simulink model "F16_Model"  (R2023b)
settings: Solver=ode4  StartTime=0.0  StopTime=inf  FixedStep=deltaTime  RelTol=1e-3
PreLoadFcn:
  | addpath(genpath(cd))
InitFcn:
  | Run_Config
undefined symbols (not defined in the file or in its folder): controlDeflections, dataBase, deltaLEF, statesFinal
libraries: simulink_extras x17, vrlib x1, sharedtransform x1
(part 2 of 2)

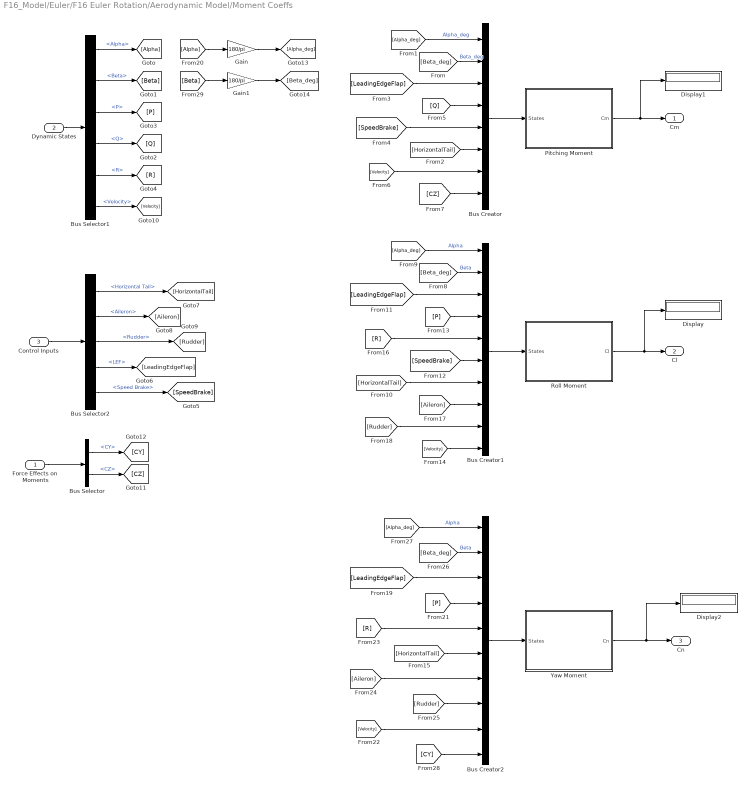
== system F16_Model/Euler/F16 Euler Rotation/Aerodynamic Model/Moment Coeffs ==
  Force Effects on Moments : Inport
  Dynamic States : Inport  Port=2
  Control Inputs : Inport  Port=3
  Bus Creator : BusCreator  Inputs=8
  Bus Creator1 : BusCreator  Inputs=10
  Bus Creator2 : BusCreator  Inputs=10
  Bus Selector : BusSelector  OutputSignals=CY,CZ
  Bus Selector1 : BusSelector  OutputSignals=Alpha,Beta,P,Q,R,Velocity
  Bus Selector2 : BusSelector  OutputSignals=Horizontal Tail,Aileron,Rudder,LEF,Speed Brake
  Display : Display
  Display1 : Display
  Display2 : Display
  Gain : Gain  Gain=180/pi
  Gain1 : Gain  Gain=180/pi
  Pitching Moment : Subsystem
  Roll Moment : Subsystem
  Yaw Moment : Subsystem
  " Cm" : Outport
  " Cl" : Outport  Port=2
  " Cn" : Outport  Port=3
  wires:
  Pitching Moment/1(Cm) -> Display1/1, " Cm"/1
  Bus Creator/1 -> Pitching Moment/1(States)
  [SpeedBrake] -> Bus Creator/5
  [LeadingEdgeFlap] -> Bus Creator/3
  [Q] -> Bus Creator/4
  [HorizontalTail] -> Bus Creator/6
  [Velocity] -> Bus Creator/7
  [CZ] -> Bus Creator/8
  Force Effects on Moments/1 -> Bus Selector/1
  Bus Selector/1 -> [CY]  "<CY>"
  Bus Selector/2 -> [CZ]  "<CZ>"
  [P] -> Bus Creator1/4
  [LeadingEdgeFlap] -> Bus Creator1/3
  Roll Moment/1(Cl) -> Display/1, " Cl"/1
  Yaw Moment/1(Cn) -> Display2/1, " Cn"/1
  [Velocity] -> Bus Creator1/10
  [R] -> Bus Creator1/5
  [SpeedBrake] -> Bus Creator1/6
  [HorizontalTail] -> Bus Creator1/7
  [Aileron] -> Bus Creator1/8
  [Rudder] -> Bus Creator1/9
  [Rudder] -> Bus Creator2/8
  [Aileron] -> Bus Creator2/7
  [HorizontalTail] -> Bus Creator2/6
  [R] -> Bus Creator2/5
  [Velocity] -> Bus Creator2/9
  [LeadingEdgeFlap] -> Bus Creator2/3
  [P] -> Bus Creator2/4
  Bus Creator2/1 -> Yaw Moment/1(States)
  Bus Selector1/4 -> [Q]  "<Q>"
  Bus Selector2/1 -> [HorizontalTail]  "<Horizontal Tail>"
  Control Inputs/1 -> Bus Selector2/1
  Bus Selector2/5 -> [SpeedBrake]  "<Speed Brake>"
  Bus Selector2/2 -> [Aileron]  "<Aileron>"
  Bus Selector1/6 -> [Velocity]  "<Velocity>"
  Bus Selector1/3 -> [P]  "<P>"
  Bus Selector1/2 -> [Beta]  "<Beta>"
  Bus Selector2/3 -> [Rudder]  "<Rudder>"
  Bus Selector1/5 -> [R]  "<R>"
  Bus Selector2/4 -> [LeadingEdgeFlap]  "<LEF>"
  Dynamic States/1 -> Bus Selector1/1
  Bus Selector1/1 -> [Alpha]  "<Alpha>"
  Bus Creator1/1 -> Roll Moment/1(States)
  Gain1/1 -> [Beta_deg]
  [Beta] -> Gain1/1
  [Alpha] -> Gain/1
  Gain/1 -> [Alpha_deg]
  [Alpha_deg] -> Bus Creator/1  "Alpha_deg"
  [Beta_deg] -> Bus Creator/2  "Beta_deg"
  [Alpha_deg] -> Bus Creator1/1  "Alpha"
  [Beta_deg] -> Bus Creator1/2  "Beta"
  [Alpha_deg] -> Bus Creator2/1  "Alpha"
  [Beta_deg] -> Bus Creator2/2  "Beta"
  [CY] -> Bus Creator2/10

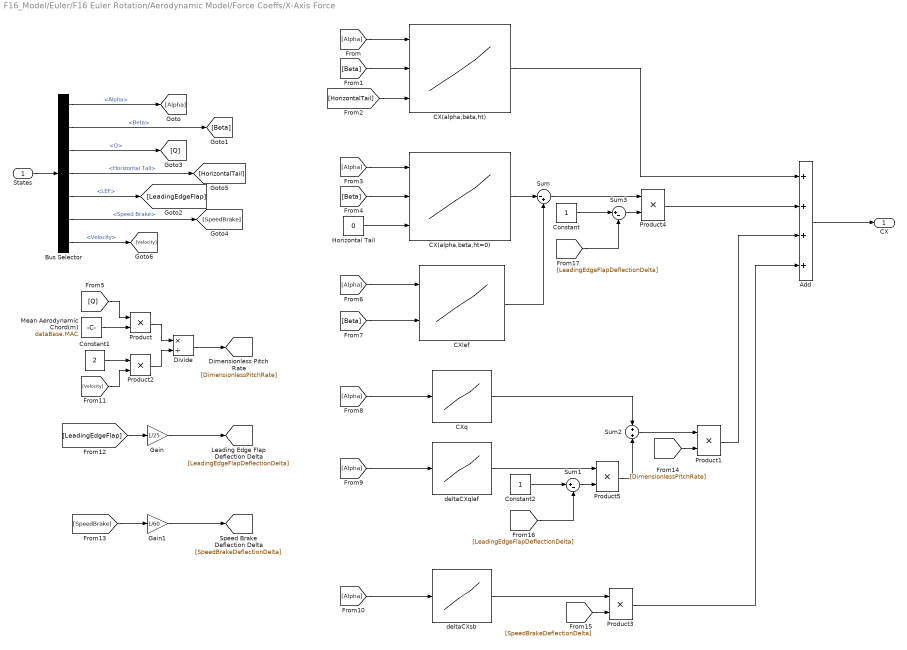
== system F16_Model/Euler/F16 Euler Rotation/Aerodynamic Model/Force Coeffs/X-Axis Force ==
  States : Inport
  Add : Sum  Inputs=++++
  Bus Selector : BusSelector  OutputSignals=Alpha,Beta,Q,Horizontal Tail,LEF,Speed Brake,Velocity
  CX(alpha,beta,ht) : Lookup_n-D  NumberOfTableDimensions=3  BreakpointsForDimension1=dataBase.f16_AerodynamicData.BP.CX.CX.alpha  BreakpointsForDimension2=dataBase.f16_AerodynamicData.BP.CX.CX.beta  BreakpointsForDimension3=dataBase.f16_AerodynamicData.BP.CX.CX.dHT  Table=dataBase.f16_AerodynamicData.data.CX.CX  InternalRulePriority=Speed  RndMeth=Simplest
      settings: InputPortMap=u0,u1,u2
  CX(alpha,beta,ht=0) : Lookup_n-D  NumberOfTableDimensions=3  BreakpointsForDimension1=dataBase.f16_AerodynamicData.BP.CX.CX.alpha  BreakpointsForDimension2=dataBase.f16_AerodynamicData.BP.CX.CX.beta  BreakpointsForDimension3=dataBase.f16_AerodynamicData.BP.CX.CX.dHT  Table=dataBase.f16_AerodynamicData.data.CX.CX  InternalRulePriority=Speed  RndMeth=Simplest
      settings: InputPortMap=u0,u1,u2
  CXlef : Lookup_n-D  BreakpointsForDimension1=dataBase.f16_AerodynamicData.BP.CX.CXlef.alpha  BreakpointsForDimension2=dataBase.f16_AerodynamicData.BP.CX.CXlef.beta  Table=dataBase.f16_AerodynamicData.data.CX.CXlef  InternalRulePriority=Speed  RndMeth=Simplest
      settings: InputPortMap=u0,u1
  CXq : Lookup_n-D  NumberOfTableDimensions=1  BreakpointsForDimension1=dataBase.f16_AerodynamicData.BP.CX.CXq.alpha  Table=dataBase.f16_AerodynamicData.data.CX.CXq  InternalRulePriority=Speed  RndMeth=Simplest
  Constant : Constant
  Constant1 : Constant  Value=2
  Constant2 : Constant
  Divide : Product  Inputs=*/
  Gain : Gain  Gain=1/25
  Gain1 : Gain  Gain=1/60
  Horizontal Tail : Constant  Value=0
  Mean Aerodynamic Chord(m) : Constant  Value=dataBase.MAC
  Product{,1..5} (6 alike) : Product
  Sum : Sum  Inputs=|-+
  Sum1 : Sum  Inputs=|+-
  Sum2 : Sum  Inputs=+|+
  Sum3 : Sum  Inputs=|+-
  deltaCXqlef : Lookup_n-D  NumberOfTableDimensions=1  BreakpointsForDimension1=dataBase.f16_AerodynamicData.BP.CX.deltaCXqlef.alpha  Table=dataBase.f16_AerodynamicData.data.CX.deltaCXqlef  InternalRulePriority=Speed  RndMeth=Simplest
  deltaCXsb : Lookup_n-D  NumberOfTableDimensions=1  BreakpointsForDimension1=dataBase.f16_AerodynamicData.BP.CX.deltaCXSB.alpha  Table=dataBase.f16_AerodynamicData.data.CX.deltaCXSB  InternalRulePriority=Speed  RndMeth=Simplest
  CX : Outport  VectorParamsAs1DForOutWhenUnconnected=off
  wires:
  States/1 -> Bus Selector/1
  [Alpha] -> CX(alpha,beta,ht)/1
  [Beta] -> CX(alpha,beta,ht)/2
  [HorizontalTail] -> CX(alpha,beta,ht)/3
  [Alpha] -> CX(alpha,beta,ht=0)/1
  Horizontal Tail/1 -> CX(alpha,beta,ht=0)/3
  [Beta] -> CX(alpha,beta,ht=0)/2
  CX(alpha,beta,ht=0)/1 -> Sum/1
  CXlef/1 -> Sum/2
  [Alpha] -> CXlef/1
  [Beta] -> CXlef/2
  [Alpha] -> CXq/1
  [Alpha] -> deltaCXqlef/1
  [Alpha] -> deltaCXsb/1
  [Q] -> Product/1
  Mean Aerodynamic Chord(m)/1 -> Product/2
  Product/1 -> Divide/1
  Divide/1 -> [DimensionlessPitchRate]
  Add/1 -> CX/1
  CX(alpha,beta,ht)/1 -> Add/1
  [LeadingEdgeFlap] -> Gain/1
  [SpeedBrake] -> Gain1/1
  Gain1/1 -> [SpeedBrakeDeflectionDelta]
  CXq/1 -> Sum2/1
  Sum2/1 -> Product1/1
  Constant1/1 -> Product2/1
  [Velocity] -> Product2/2
  Product2/1 -> Divide/2
  [DimensionlessPitchRate] -> Product1/2
  deltaCXsb/1 -> Product3/1
  [SpeedBrakeDeflectionDelta] -> Product3/2
  Product1/1 -> Add/3
  Product3/1 -> Add/4
  Sum/1 -> Product4/1
  Product4/1 -> Add/2
  Gain/1 -> [LeadingEdgeFlapDeflectionDelta]
  Constant/1 -> Sum3/1
  Sum3/1 -> Product4/2
  [LeadingEdgeFlapDeflectionDelta] -> Sum3/2
  [LeadingEdgeFlapDeflectionDelta] -> Sum1/2
  Constant2/1 -> Sum1/1
  Product5/1 -> Sum2/2
  deltaCXqlef/1 -> Product5/1
  Sum1/1 -> Product5/2
  Bus Selector/1 -> [Alpha]  "<Alpha>"
  Bus Selector/2 -> [Beta]  "<Beta>"
  Bus Selector/3 -> [Q]  "<Q>"
  Bus Selector/4 -> [HorizontalTail]  "<Horizontal Tail>"
  Bus Selector/5 -> [LeadingEdgeFlap]  "<LEF>"
  Bus Selector/6 -> [SpeedBrake]  "<Speed Brake>"
  Bus Selector/7 -> [Velocity]  "<Velocity>"

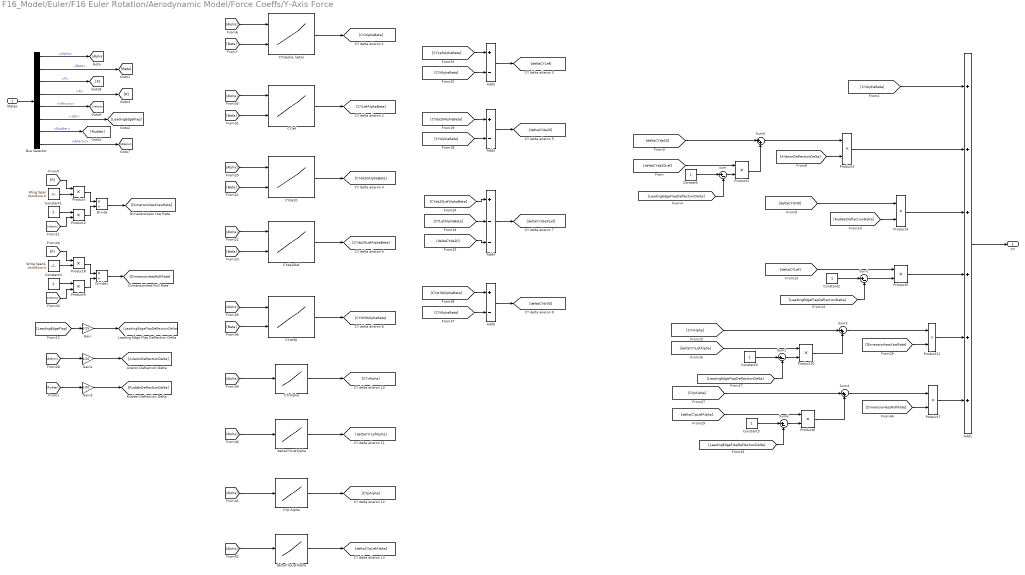
== system F16_Model/Euler/F16 Euler Rotation/Aerodynamic Model/Force Coeffs/Y-Axis Force ==
  States : Inport
  Add1 : Sum  Inputs=++++++
  Add2 : Sum  Inputs=+-
  Add3 : Sum  Inputs=+-
  Add4 : Sum  Inputs=+--
  Add5 : Sum  Inputs=+-
  Bus Selector : BusSelector  OutputSignals=Alpha,Beta,P,R,Velocity,LEF,Rudder,Aileron
  "CY(alpha, beta)" : Lookup_n-D  BreakpointsForDimension1=dataBase.f16_AerodynamicData.BP.CY.CY.alpha  BreakpointsForDimension2=dataBase.f16_AerodynamicData.BP.CY.CY.beta  Table=dataBase.f16_AerodynamicData.data.CY.CY  InternalRulePriority=Speed  RndMeth=Simplest
      settings: InputPortMap=u0,u1
  CYda20 : Lookup_n-D  BreakpointsForDimension1=dataBase.f16_AerodynamicData.BP.CY.CYda20.alpha  BreakpointsForDimension2=dataBase.f16_AerodynamicData.BP.CY.CYda20.beta  Table=dataBase.f16_AerodynamicData.data.CY.CYda20  InternalRulePriority=Speed  RndMeth=Simplest
      settings: InputPortMap=u0,u1
  CYda20lef : Lookup_n-D  BreakpointsForDimension1=dataBase.f16_AerodynamicData.BP.CY.CYda20lef.alpha  BreakpointsForDimension2=dataBase.f16_AerodynamicData.BP.CY.CYda20lef.beta  Table=dataBase.f16_AerodynamicData.data.CY.CYda20lef  InternalRulePriority=Speed  RndMeth=Simplest
      settings: InputPortMap=u0,u1
  CYdr30 : Lookup_n-D  BreakpointsForDimension1=dataBase.f16_AerodynamicData.BP.CY.CYdr30.alpha  BreakpointsForDimension2=dataBase.f16_AerodynamicData.BP.CY.CYdr30.beta  Table=dataBase.f16_AerodynamicData.data.CY.CYdr30  InternalRulePriority=Speed  RndMeth=Simplest
      settings: InputPortMap=u0,u1
  CYlef : Lookup_n-D  BreakpointsForDimension1=dataBase.f16_AerodynamicData.BP.CY.CYlef.alpha  BreakpointsForDimension2=dataBase.f16_AerodynamicData.BP.CY.CYlef.beta  Table=dataBase.f16_AerodynamicData.data.CY.CYlef  InternalRulePriority=Speed  RndMeth=Simplest
      settings: InputPortMap=u0,u1
  CYp Alpha : Lookup_n-D  NumberOfTableDimensions=1  BreakpointsForDimension1=dataBase.f16_AerodynamicData.BP.CY.CYp.alpha  Table=dataBase.f16_AerodynamicData.data.CY.CYp  InternalRulePriority=Speed  RndMeth=Simplest
  CYrAlpha : Lookup_n-D  NumberOfTableDimensions=1  BreakpointsForDimension1=dataBase.f16_AerodynamicData.BP.CY.CYr.alpha  Table=dataBase.f16_AerodynamicData.data.CY.CYr  InternalRulePriority=Speed  RndMeth=Simplest
  Constant{,2..3,5} (4 alike) : Constant
  Constant1 : Constant  Value=2
  Constant4 : Constant  Value=2
  Divide : Product  Inputs=*/
  Divide1 : Product  Inputs=*/
  Gain : Gain  Gain=1/25
  Gain2 : Gain  Gain=1/20
  Gain3 : Gain  Gain=1/30
  Product{,1..11} (12 alike) : Product
  Sum{,1..2,6} (4 alike) : Sum  Inputs=|+-
  Sum3 : Sum  Inputs=|++
  Sum4 : Sum  Inputs=|++
  Sum5 : Sum  Inputs=|++
  Wing Span : Constant  Value=dataBase.b
  Wing Span1 : Constant  Value=dataBase.b
  deltaCYpLefAlpha : Lookup_n-D  NumberOfTableDimensions=1  BreakpointsForDimension1=dataBase.f16_AerodynamicData.BP.CY.deltaCYplef.alpha  Table=dataBase.f16_AerodynamicData.data.CY.deltaCYplef  InternalRulePriority=Speed  RndMeth=Simplest
  deltaCYrLefAlpha : Lookup_n-D  NumberOfTableDimensions=1  BreakpointsForDimension1=dataBase.f16_AerodynamicData.BP.CY.deltaCYrlef.alpha  Table=dataBase.f16_AerodynamicData.data.CY.deltaCYrlef  InternalRulePriority=Speed  RndMeth=Simplest
  CY : Outport  VectorParamsAs1DForOutWhenUnconnected=off
  wires:
  Wing Span/1 -> Product/2
  Divide/1 -> [DimensionlessYawRate]
  [LeadingEdgeFlap] -> Gain/1
  Constant1/1 -> Product2/1
  [Beta] -> "CY(alpha, beta)"/2
  [R] -> Product/1
  States/1 -> Bus Selector/1
  Product2/1 -> Divide/2
  Product/1 -> Divide/1
  [Alpha] -> "CY(alpha, beta)"/1
  Gain/1 -> [LeadingEdgeFlapDeflectionDelta]
  [Velocity] -> Product2/2
  Add1/1 -> CY/1
  "CY(alpha, beta)"/1 -> [CYAlphaBeta]
  [Beta] -> CYda20/2
  [Alpha] -> CYda20/1
  [Alpha] -> CYda20lef/1
  [Beta] -> CYda20lef/2
  [Aileron] -> Gain2/1
  Gain2/1 -> [AileronDeflectionDelta]
  [Alpha] -> CYlef/1
  [Beta] -> CYlef/2
  CYlef/1 -> [CYLefAlphaBeta]
  Add2/1 -> [deltaCYLef]
  [CYAlphaBeta] -> Add2/2
  [CYLefAlphaBeta] -> Add2/1
  CYda20/1 -> [CYda20AlphaBeta]
  [CYda20AlphaBeta] -> Add3/1
  [CYAlphaBeta] -> Add3/2
  Add3/1 -> [deltaCYda20]
  CYda20lef/1 -> [CYda20LefAlphaBeta]
  [CYda20LefAlphaBeta] -> Add4/1
  [CYLefAlphaBeta] -> Add4/2
  [deltaCYda20] -> Add4/3
  Add4/1 -> [deltaCYda20Lef]
  CYdr30/1 -> [CYdr30AlphaBeta]
  [Alpha] -> CYdr30/1
  [Beta] -> CYdr30/2
  Add5/1 -> [deltaCYdr30]
  [CYAlphaBeta] -> Add5/2
  [CYdr30AlphaBeta] -> Add5/1
  [Alpha] -> CYrAlpha/1
  CYrAlpha/1 -> [CYrAlpha]
  deltaCYrLefAlpha/1 -> [deltaCYrLefAlpha]
  [Alpha] -> deltaCYrLefAlpha/1
  [Alpha] -> deltaCYpLefAlpha/1
  deltaCYpLefAlpha/1 -> [deltaCYpLefAlpha]
  CYp Alpha/1 -> [CYpAlpha]
  [Alpha] -> CYp Alpha/1
  [Velocity] -> Product9/2
  Product8/1 -> Divide1/1
  Product9/1 -> Divide1/2
  [P] -> Product8/1
  Constant4/1 -> Product9/1
  Divide1/1 -> [DimensionlessRollRate]
  Wing Span1/1 -> Product8/2
  Gain3/1 -> [RudderDeflectionDelta]
  [Rudder] -> Gain3/1
  [CYAlphaBeta] -> Add1/1
  [deltaCYda20Lef] -> Product1/1
  [deltaCYda20] -> Sum5/1
  Product1/1 -> Sum5/2
  Sum5/1 -> Product3/1
  [AileronDeflectionDelta] -> Product3/2
  Product3/1 -> Add1/2
  [RudderDeflectionDelta] -> Product4/2
  [deltaCYdr30] -> Product4/1
  Product4/1 -> Add1/3
  [deltaCYLef] -> Product5/1
  Product5/1 -> Add1/4
  [CYrAlpha] -> Sum3/1
  [deltaCYrLefAlpha] -> Product10/1
  Product10/1 -> Sum3/2
  [DimensionlessYawRate] -> Product11/2
  Sum3/1 -> Product11/1
  Product11/1 -> Add1/5
  Product7/1 -> Add1/6
  Sum4/1 -> Product7/1
  [DimensionlessRollRate] -> Product7/2
  Product6/1 -> Sum4/2
  [deltaCYpLefAlpha] -> Product6/1
  [CYpAlpha] -> Sum4/1
  Constant/1 -> Sum/1
  [LeadingEdgeFlapDeflectionDelta] -> Sum/2
  Sum/1 -> Product1/2
  Constant2/1 -> Sum1/1
  [LeadingEdgeFlapDeflectionDelta] -> Sum1/2
  Sum1/1 -> Product5/2
  Constant3/1 -> Sum2/1
  [LeadingEdgeFlapDeflectionDelta] -> Sum2/2
  Sum2/1 -> Product10/2
  Constant5/1 -> Sum6/1
  [LeadingEdgeFlapDeflectionDelta] -> Sum6/2
  Sum6/1 -> Product6/2
  Bus Selector/1 -> [Alpha]  "<Alpha>"
  Bus Selector/2 -> [Beta]  "<Beta>"
  Bus Selector/3 -> [P]  "<P>"
  Bus Selector/4 -> [R]  "<R>"
  Bus Selector/5 -> [Velocity]  "<Velocity>"
  Bus Selector/6 -> [LeadingEdgeFlap]  "<LEF>"
  Bus Selector/7 -> [Rudder]  "<Rudder>"
  Bus Selector/8 -> [Aileron]  "<Aileron>"

== system F16_Model/Euler/F16 Euler Rotation/Aerodynamic Model/Force Coeffs/Z-Axis Force ==
  States : Inport
  Add : Sum  Inputs=++++
  Bus Selector : BusSelector  OutputSignals=Alpha,Beta,Q,Horizontal Tail,LEF,Speed Brake,Velocity
  CZ(alpha,beta,ht) : Lookup_n-D  NumberOfTableDimensions=3  BreakpointsForDimension1=dataBase.f16_AerodynamicData.BP.CZ.CZ.alpha  BreakpointsForDimension2=dataBase.f16_AerodynamicData.BP.CZ.CZ.beta  BreakpointsForDimension3=dataBase.f16_AerodynamicData.BP.CZ.CZ.dHT  Table=dataBase.f16_AerodynamicData.data.CZ.CZ  InternalRulePriority=Speed  RndMeth=Simplest
      settings: InputPortMap=u0,u1,u2
  CZ(alpha,beta,ht=0) : Lookup_n-D  NumberOfTableDimensions=3  BreakpointsForDimension1=dataBase.f16_AerodynamicData.BP.CZ.CZ.alpha  BreakpointsForDimension2=dataBase.f16_AerodynamicData.BP.CZ.CZ.beta  BreakpointsForDimension3=dataBase.f16_AerodynamicData.BP.CZ.CZ.dHT  Table=dataBase.f16_AerodynamicData.data.CZ.CZ  InternalRulePriority=Speed  RndMeth=Simplest
      settings: InputPortMap=u0,u1,u2
  CZlef : Lookup_n-D  BreakpointsForDimension1=dataBase.f16_AerodynamicData.BP.CZ.CZlef.alpha  BreakpointsForDimension2=dataBase.f16_AerodynamicData.BP.CZ.CZlef.beta  Table=dataBase.f16_AerodynamicData.data.CZ.CZlef  InternalRulePriority=Speed  RndMeth=Simplest
      settings: InputPortMap=u0,u1
  CZq : Lookup_n-D  NumberOfTableDimensions=1  BreakpointsForDimension1=dataBase.f16_AerodynamicData.BP.CZ.CZq.alpha  Table=dataBase.f16_AerodynamicData.data.CZ.CZq  InternalRulePriority=Speed  RndMeth=Simplest
  Constant : Constant
  Constant1 : Constant  Value=2
  Constant2 : Constant
  Divide : Product  Inputs=*/
  Gain : Gain  Gain=1/25
  Gain1 : Gain  Gain=1/60
  Horizontal Tail : Constant  Value=0
  Mean Aerodynamic Chord(m) : Constant  Value=dataBase.MAC
  Product{,1..5} (6 alike) : Product
  Sum : Sum  Inputs=|-+
  Sum1 : Sum  Inputs=|+-
  Sum2 : Sum  Inputs=+|+
  Sum3 : Sum  Inputs=|+-
  deltaCZqlef : Lookup_n-D  NumberOfTableDimensions=1  BreakpointsForDimension1=dataBase.f16_AerodynamicData.BP.CZ.deltaCZqlef.alpha  Table=dataBase.f16_AerodynamicData.data.CZ.deltaCZqlef  InternalRulePriority=Speed  RndMeth=Simplest
  deltaCZsb : Lookup_n-D  NumberOfTableDimensions=1  BreakpointsForDimension1=dataBase.f16_AerodynamicData.BP.CZ.deltaCZSB.alpha  Table=dataBase.f16_AerodynamicData.data.CZ.deltaCZSB  InternalRulePriority=Speed  RndMeth=Simplest
  CZ : Outport  VectorParamsAs1DForOutWhenUnconnected=off
  wires:
  [Beta] -> CZ(alpha,beta,ht=0)/2
  Product2/1 -> Divide/2
  [Alpha] -> CZlef/1
  [Velocity] -> Product2/2
  Sum2/1 -> Product1/1
  [SpeedBrake] -> Gain1/1
  Product/1 -> Divide/1
  [LeadingEdgeFlap] -> Gain/1
  Divide/1 -> [DimensionlessPitchRate]
  Mean Aerodynamic Chord(m)/1 -> Product/2
  [Alpha] -> deltaCZsb/1
  [HorizontalTail] -> CZ(alpha,beta,ht)/3
  CZlef/1 -> Sum/2
  Constant1/1 -> Product2/1
  [Beta] -> CZ(alpha,beta,ht)/2
  Horizontal Tail/1 -> CZ(alpha,beta,ht=0)/3
  [Alpha] -> CZ(alpha,beta,ht=0)/1
  [Alpha] -> CZq/1
  [Alpha] -> deltaCZqlef/1
  [Alpha] -> CZ(alpha,beta,ht)/1
  States/1 -> Bus Selector/1
  CZ(alpha,beta,ht=0)/1 -> Sum/1
  Sum/1 -> Product4/1
  Product3/1 -> Add/4
  CZq/1 -> Sum2/1
  Gain1/1 -> [SpeedBrakeDeflectionDelta]
  CZ(alpha,beta,ht)/1 -> Add/1
  Add/1 -> CZ/1
  deltaCZsb/1 -> Product3/1
  [SpeedBrakeDeflectionDelta] -> Product3/2
  [Q] -> Product/1
  [DimensionlessPitchRate] -> Product1/2
  [Beta] -> CZlef/2
  Product1/1 -> Add/3
  Gain/1 -> [LeadingEdgeFlapDeflectionDelta]
  Product4/1 -> Add/2
  deltaCZqlef/1 -> Product5/1
  Product5/1 -> Sum2/2
  Sum3/1 -> Product4/2
  [LeadingEdgeFlapDeflectionDelta] -> Sum3/2
  Constant/1 -> Sum3/1
  Sum1/1 -> Product5/2
  [LeadingEdgeFlapDeflectionDelta] -> Sum1/2
  Constant2/1 -> Sum1/1
  Bus Selector/1 -> [Alpha]  "<Alpha>"
  Bus Selector/2 -> [Beta]  "<Beta>"
  Bus Selector/3 -> [Q]  "<Q>"
  Bus Selector/4 -> [HorizontalTail]  "<Horizontal Tail>"
  Bus Selector/5 -> [LeadingEdgeFlap]  "<LEF>"
  Bus Selector/7 -> [Velocity]  "<Velocity>"
  Bus Selector/6 -> [SpeedBrake]  "<Speed Brake>"

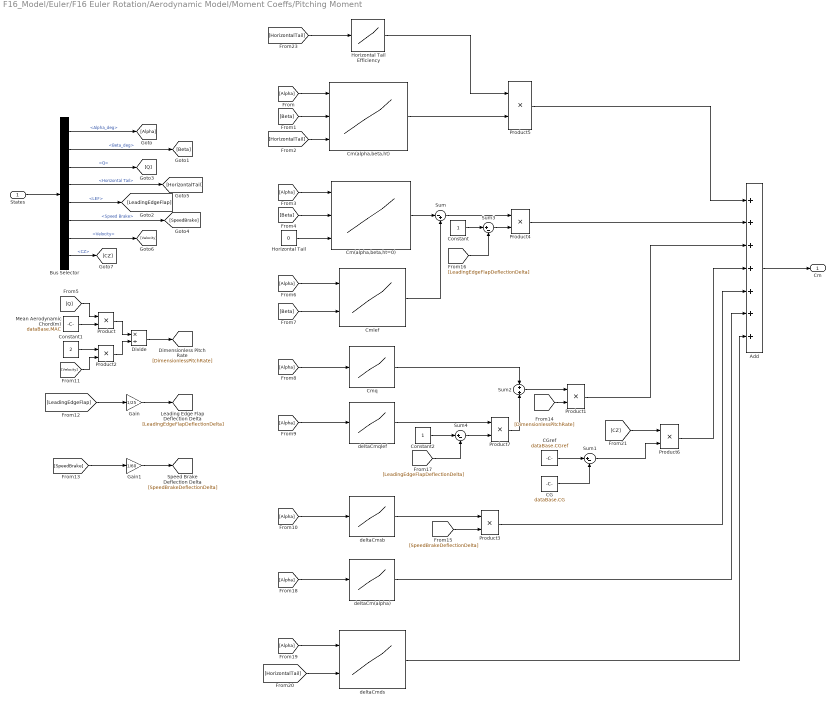
== system F16_Model/Euler/F16 Euler Rotation/Aerodynamic Model/Moment Coeffs/Pitching Moment ==
  States : Inport
  Add : Sum  Inputs=+++++++
  Bus Selector : BusSelector  OutputSignals=Alpha_deg,Beta_deg,Q,Horizontal Tail,LEF,Speed Brake,Velocity,CZ
  CG : Constant  Value=dataBase.CG
  CGref : Constant  Value=dataBase.CGref
  Cm(alpha,beta,ht) : Lookup_n-D  NumberOfTableDimensions=3  BreakpointsForDimension1=dataBase.f16_AerodynamicData.BP.Cm.Cm.alpha  BreakpointsForDimension2=dataBase.f16_AerodynamicData.BP.Cm.Cm.beta  BreakpointsForDimension3=dataBase.f16_AerodynamicData.BP.Cm.Cm.dHT  Table=dataBase.f16_AerodynamicData.data.Cm.Cm  ExtrapMethod=Clip  InternalRulePriority=Speed  RndMeth=Simplest
      settings: InputPortMap=u0,u1,u2
  Cm(alpha,beta,ht=0) : Lookup_n-D  NumberOfTableDimensions=3  BreakpointsForDimension1=dataBase.f16_AerodynamicData.BP.Cm.Cm.alpha  BreakpointsForDimension2=dataBase.f16_AerodynamicData.BP.Cm.Cm.beta  BreakpointsForDimension3=dataBase.f16_AerodynamicData.BP.Cm.Cm.dHT  Table=dataBase.f16_AerodynamicData.data.Cm.Cm  ExtrapMethod=Clip  InternalRulePriority=Speed  RndMeth=Simplest
      settings: InputPortMap=u0,u1,u2
  Cmlef : Lookup_n-D  BreakpointsForDimension1=dataBase.f16_AerodynamicData.BP.Cm.Cmlef.alpha  BreakpointsForDimension2=dataBase.f16_AerodynamicData.BP.Cm.Cmlef.beta  Table=dataBase.f16_AerodynamicData.data.Cm.Cmlef  ExtrapMethod=Clip  InternalRulePriority=Speed  RndMeth=Simplest
      settings: InputPortMap=u0,u1
  Cmq : Lookup_n-D  NumberOfTableDimensions=1  BreakpointsForDimension1=dataBase.f16_AerodynamicData.BP.Cm.Cmq.alpha  Table=dataBase.f16_AerodynamicData.data.Cm.Cmq  ExtrapMethod=Clip  InternalRulePriority=Speed  RndMeth=Simplest
  Constant : Constant
  Constant1 : Constant  Value=2
  Constant2 : Constant
  Divide : Product  Inputs=*/
  Gain : Gain  Gain=1/25
  Gain1 : Gain  Gain=1/60
  Horizontal Tail : Constant  Value=0
  Horizontal Tail Efficiency : Lookup_n-D  NumberOfTableDimensions=1  BreakpointsForDimension1=dataBase.f16_AerodynamicData.BP.Cm.n_dHT.dHT  Table=dataBase.f16_AerodynamicData.data.Cm.n_dHT  ExtrapMethod=Clip  InternalRulePriority=Speed  RndMeth=Simplest
  Mean Aerodynamic Chord(m) : Constant  Value=dataBase.MAC
  Product{,1..7} (8 alike) : Product
  Sum : Sum  Inputs=|-+
  Sum1 : Sum  Inputs=|+-
  Sum2 : Sum  Inputs=+|+
  Sum3 : Sum  Inputs=|+-
  Sum4 : Sum  Inputs=|+-
  deltaCm(alpha) : Lookup_n-D  NumberOfTableDimensions=1  BreakpointsForDimension1=dataBase.f16_AerodynamicData.BP.Cm.deltaCm.alpha  Table=dataBase.f16_AerodynamicData.data.Cm.deltaCm  ExtrapMethod=Clip  InternalRulePriority=Speed  RndMeth=Simplest
  deltaCmds : Lookup_n-D  BreakpointsForDimension1=dataBase.f16_AerodynamicData.BP.Cm.deltaCmds.alpha  BreakpointsForDimension2=dataBase.f16_AerodynamicData.BP.Cm.deltaCmds.dHT  Table=dataBase.f16_AerodynamicData.data.Cm.deltaCmds  ExtrapMethod=Clip  InternalRulePriority=Speed  RndMeth=Simplest
      settings: InputPortMap=u0,u1
  deltaCmqlef : Lookup_n-D  NumberOfTableDimensions=1  BreakpointsForDimension1=dataBase.f16_AerodynamicData.BP.Cm.deltaCmqlef.alpha  Table=dataBase.f16_AerodynamicData.data.Cm.deltaCmqlef  ExtrapMethod=Clip  InternalRulePriority=Speed  RndMeth=Simplest
  deltaCmsb : Lookup_n-D  NumberOfTableDimensions=1  BreakpointsForDimension1=dataBase.f16_AerodynamicData.BP.Cm.deltaCmSB.alpha  Table=dataBase.f16_AerodynamicData.data.Cm.deltaCmSB  ExtrapMethod=Clip  InternalRulePriority=Speed  RndMeth=Simplest
  Cm : Outport
  wires:
  [Beta] -> Cm(alpha,beta,ht=0)/2
  [SpeedBrakeDeflectionDelta] -> Product3/2
  Constant1/1 -> Product2/1
  [Alpha] -> Cm(alpha,beta,ht=0)/1
  Product/1 -> Divide/1
  Cm(alpha,beta,ht=0)/1 -> Sum/1
  Horizontal Tail/1 -> Cm(alpha,beta,ht=0)/3
  [Alpha] -> Cm(alpha,beta,ht)/1
  States/1 -> Bus Selector/1
  [Alpha] -> Cmlef/1
  [Alpha] -> deltaCmqlef/1
  [Alpha] -> Cmq/1
  Mean Aerodynamic Chord(m)/1 -> Product/2
  Product1/1 -> Add/3
  Sum2/1 -> Product1/1
  [Q] -> Product/1
  Gain1/1 -> [SpeedBrakeDeflectionDelta]
  Cmlef/1 -> Sum/2
  [DimensionlessPitchRate] -> Product1/2
  [Beta] -> Cm(alpha,beta,ht)/2
  Divide/1 -> [DimensionlessPitchRate]
  Product4/1 -> Add/2
  Add/1 -> Cm/1
  [LeadingEdgeFlap] -> Gain/1
  [HorizontalTail] -> Cm(alpha,beta,ht)/3
  [SpeedBrake] -> Gain1/1
  Product2/1 -> Divide/2
  Gain/1 -> [LeadingEdgeFlapDeflectionDelta]
  [Velocity] -> Product2/2
  deltaCmsb/1 -> Product3/1
  Sum/1 -> Product4/1
  [Alpha] -> deltaCmsb/1
  Cmq/1 -> Sum2/1
  [Beta] -> Cmlef/2
  [Alpha] -> deltaCm(alpha)/1
  [HorizontalTail] -> deltaCmds/2
  [Alpha] -> deltaCmds/1
  Product5/1 -> Add/1
  [CZ] -> Product6/1
  CGref/1 -> Sum1/1
  CG/1 -> Sum1/2
  deltaCmqlef/1 -> Product7/1
  Product7/1 -> Sum2/2
  [HorizontalTail] -> Horizontal Tail Efficiency/1
  Cm(alpha,beta,ht)/1 -> Product5/2
  Horizontal Tail Efficiency/1 -> Product5/1
  Constant/1 -> Sum3/1
  [LeadingEdgeFlapDeflectionDelta] -> Sum3/2
  Sum3/1 -> Product4/2
  Constant2/1 -> Sum4/1
  Sum4/1 -> Product7/2
  [LeadingEdgeFlapDeflectionDelta] -> Sum4/2
  Product6/1 -> Add/4
  Product3/1 -> Add/5
  deltaCm(alpha)/1 -> Add/6
  deltaCmds/1 -> Add/7
  Bus Selector/1 -> [Alpha]  "<Alpha_deg>"
  Bus Selector/2 -> [Beta]  "<Beta_deg>"
  Bus Selector/3 -> [Q]  "<Q>"
  Bus Selector/4 -> [HorizontalTail]  "<Horizontal Tail>"
  Bus Selector/5 -> [LeadingEdgeFlap]  "<LEF>"
  Bus Selector/6 -> [SpeedBrake]  "<Speed Brake>"
  Bus Selector/7 -> [Velocity]  "<Velocity>"
  Bus Selector/8 -> [CZ]  "<CZ>"
  Sum1/1 -> Product6/2

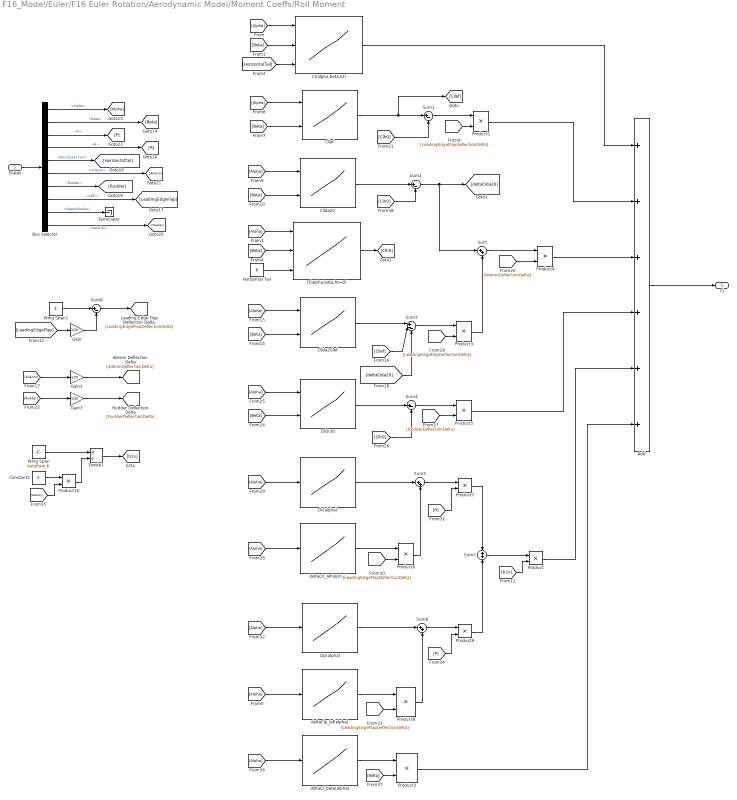
== system F16_Model/Euler/F16 Euler Rotation/Aerodynamic Model/Moment Coeffs/Roll Moment ==
  States : Inport
  Add : Sum  Inputs=++++++
  Bus Selector : BusSelector  OutputSignals=Alpha,Beta,P,R,Horizontal Tail,Aileron,Rudder,LEF,Speed Brake,Velocity
  Cl(alpha,beta,ht) : Lookup_n-D  NumberOfTableDimensions=3  BreakpointsForDimension1=dataBase.f16_AerodynamicData.BP.Cl.Cl.alpha  BreakpointsForDimension2=dataBase.f16_AerodynamicData.BP.Cl.Cl.beta  BreakpointsForDimension3=dataBase.f16_AerodynamicData.BP.Cl.Cl.dHT  Table=dataBase.f16_AerodynamicData.data.Cl.Cl  ExtrapMethod=Clip  InternalRulePriority=Speed  RndMeth=Simplest
      settings: InputPortMap=u0,u1,u2
  Cl(alpha,beta,ht=0) : Lookup_n-D  NumberOfTableDimensions=3  BreakpointsForDimension1=dataBase.f16_AerodynamicData.BP.Cl.Cl.alpha  BreakpointsForDimension2=dataBase.f16_AerodynamicData.BP.Cl.Cl.beta  BreakpointsForDimension3=dataBase.f16_AerodynamicData.BP.Cl.Cl.dHT  Table=dataBase.f16_AerodynamicData.data.Cl.Cl  ExtrapMethod=Clip  InternalRulePriority=Speed  RndMeth=Simplest
      settings: InputPortMap=u0,u1,u2
  Cllda20 : Lookup_n-D  BreakpointsForDimension1=dataBase.f16_AerodynamicData.BP.Cl.Clda20.alpha  BreakpointsForDimension2=dataBase.f16_AerodynamicData.BP.Cl.Clda20.beta  Table=dataBase.f16_AerodynamicData.data.Cl.Clda20  ExtrapMethod=Clip  InternalRulePriority=Speed  RndMeth=Simplest
      settings: InputPortMap=u0,u1
  Cllda20lef : Lookup_n-D  BreakpointsForDimension1=dataBase.f16_AerodynamicData.BP.Cl.Clda20lef.alpha  BreakpointsForDimension2=dataBase.f16_AerodynamicData.BP.Cl.Clda20lef.beta  Table=dataBase.f16_AerodynamicData.data.Cl.Clda20lef  ExtrapMethod=Clip  InternalRulePriority=Speed  RndMeth=Simplest
      settings: InputPortMap=u0,u1
  Clldr30 : Lookup_n-D  BreakpointsForDimension1=dataBase.f16_AerodynamicData.BP.Cl.Cldr30.alpha  BreakpointsForDimension2=dataBase.f16_AerodynamicData.BP.Cl.Cldr30.beta  Table=dataBase.f16_AerodynamicData.data.Cl.Cldr30  ExtrapMethod=Clip  InternalRulePriority=Speed  RndMeth=Simplest
      settings: InputPortMap=u0,u1
  Cllef : Lookup_n-D  BreakpointsForDimension1=dataBase.f16_AerodynamicData.BP.Cl.Cllef.alpha  BreakpointsForDimension2=dataBase.f16_AerodynamicData.BP.Cl.Cllef.beta  Table=dataBase.f16_AerodynamicData.data.Cl.Cllef  ExtrapMethod=Clip  InternalRulePriority=Speed  RndMeth=Simplest
      settings: InputPortMap=u0,u1
  Clp(alpha) : Lookup_n-D  NumberOfTableDimensions=1  BreakpointsForDimension1=dataBase.f16_AerodynamicData.BP.Cl.Clp.alpha  BreakpointsForDimension2=dataBase.f16_AerodynamicData.BP.Cl.Cldr30.beta  Table=dataBase.f16_AerodynamicData.data.Cl.Clp  ExtrapMethod=Clip  InternalRulePriority=Speed  RndMeth=Simplest
  Clr(alpha) : Lookup_n-D  NumberOfTableDimensions=1  BreakpointsForDimension1=dataBase.f16_AerodynamicData.BP.Cl.Clr.alpha  BreakpointsForDimension2=dataBase.f16_AerodynamicData.BP.Cl.Cldr30.beta  Table=dataBase.f16_AerodynamicData.data.Cl.Clr  ExtrapMethod=Clip  InternalRulePriority=Speed  RndMeth=Simplest
  Constant2 : Constant  Value=2
  Divide1 : Product  Inputs=*/
  Gain : Gain  Gain=1/25
  Gain2 : Gain  Gain=1/20
  Gain3 : Gain  Gain=1/30
  Horizontal Tail : Constant  Value=0
  Product{,1..10} (11 alike) : Product
  Sum : Sum  Inputs=|++
  Sum{1..2,4,8} (4 alike) : Sum  Inputs=|+-
  Sum3 : Sum  Inputs=|+--
  Sum5 : Sum  Inputs=|++
  Sum6 : Sum  Inputs=|++
  Sum7 : Sum  Inputs=+|+
  Terminator : Terminator
  Wing Span : Constant  Value=dataBase.b
  Wing Span1 : Constant
  deltaCl_beta(alpha) : Lookup_n-D  NumberOfTableDimensions=1  BreakpointsForDimension1=dataBase.f16_AerodynamicData.BP.Cl.deltaClBeta.alpha  BreakpointsForDimension2=dataBase.f16_AerodynamicData.BP.Cl.Cldr30.beta  Table=dataBase.f16_AerodynamicData.data.Cl.deltaClBeta  ExtrapMethod=Clip  InternalRulePriority=Speed  RndMeth=Simplest
  deltaClp_lef(alpha) : Lookup_n-D  NumberOfTableDimensions=1  BreakpointsForDimension1=dataBase.f16_AerodynamicData.BP.Cl.deltaClplef.alpha  BreakpointsForDimension2=dataBase.f16_AerodynamicData.BP.Cl.Cldr30.beta  Table=dataBase.f16_AerodynamicData.data.Cl.deltaClplef  ExtrapMethod=Clip  InternalRulePriority=Speed  RndMeth=Simplest
  deltaClr_lef(alpha) : Lookup_n-D  NumberOfTableDimensions=1  BreakpointsForDimension1=dataBase.f16_AerodynamicData.BP.Cl.deltaClrlef.alpha  BreakpointsForDimension2=dataBase.f16_AerodynamicData.BP.Cl.Cldr30.beta  Table=dataBase.f16_AerodynamicData.data.Cl.deltaClrlef  ExtrapMethod=Clip  InternalRulePriority=Speed  RndMeth=Simplest
  Cl : Outport
  wires:
  [Beta] -> Cllef/2
  [HorizontalTail] -> Cl(alpha,beta,ht)/3
  Cl(alpha,beta,ht)/1 -> Add/1
  [Alpha] -> Cllef/1
  [Alpha] -> Cl(alpha,beta,ht)/1
  [Beta] -> Cl(alpha,beta,ht)/2
  Add/1 -> Cl/1
  Gain/1 -> Sum8/2
  [LeadingEdgeFlap] -> Gain/1
  [Aileron] -> Gain2/1
  Gain2/1 -> [AileronDeflectionDelta]
  Gain3/1 -> [RudderDeflectionDelta]
  [Rudder] -> Gain3/1
  [Beta] -> Cl(alpha,beta,ht=0)/2
  Horizontal Tail/1 -> Cl(alpha,beta,ht=0)/3
  [Alpha] -> Cl(alpha,beta,ht=0)/1
  Cllef/1 -> Sum1/1, [Cllef]
  [LeadingEdgeFlapDeflectionDelta] -> Product1/2
  Sum1/1 -> Product1/1
  Cl(alpha,beta,ht=0)/1 -> [Clh0]
  [Beta] -> Cllda20/2
  [Alpha] -> Cllda20/1
  Cllda20/1 -> Sum2/1
  Product1/1 -> Add/2
  Sum2/1 -> Sum/1, [deltaClda20]
  [Alpha] -> Cllda20lef/1
  [Beta] -> Cllda20lef/2
  Cllda20lef/1 -> Sum3/1
  [Cllef] -> Sum3/2
  [deltaClda20] -> Sum3/3
  [LeadingEdgeFlapDeflectionDelta] -> Product3/2
  Sum3/1 -> Product3/1
  Product3/1 -> Sum/2
  [AileronDeflectionDelta] -> Product4/2
  Sum/1 -> Product4/1
  Product4/1 -> Add/3
  [Clh0] -> Sum1/2
  [Clh0] -> Sum2/2
  [Alpha] -> Clldr30/1
  [Beta] -> Clldr30/2
  Clldr30/1 -> Sum4/1
  [Clh0] -> Sum4/2
  [RudderDeflectionDelta] -> Product5/2
  Sum4/1 -> Product5/1
  Product5/1 -> Add/4
  [Alpha] -> Clr(alpha)/1
  Clr(alpha)/1 -> Sum5/1
  [Alpha] -> deltaClr_lef(alpha)/1
  [LeadingEdgeFlapDeflectionDelta] -> Product6/2
  deltaClr_lef(alpha)/1 -> Product6/1
  Product6/1 -> Sum5/2
  [Alpha] -> Clp(alpha)/1
  [Alpha] -> deltaClp_lef(alpha)/1
  [LeadingEdgeFlapDeflectionDelta] -> Product8/2
  deltaClp_lef(alpha)/1 -> Product8/1
  Product8/1 -> Sum6/2
  Clp(alpha)/1 -> Sum6/1
  Sum6/1 -> Product9/1
  [P] -> Product9/2
  Sum5/1 -> Product7/1
  [R] -> Product7/2
  Product7/1 -> Sum7/1
  Product9/1 -> Sum7/2
  [Velocity] -> Product10/2
  Constant2/1 -> Product10/1
  Product10/1 -> Divide1/2
  Wing Span/1 -> Divide1/1
  Divide1/1 -> [b2v]
  Sum7/1 -> Product/1
  [b2v] -> Product/2
  [Alpha] -> deltaCl_beta(alpha)/1
  deltaCl_beta(alpha)/1 -> Product2/1
  [Beta] -> Product2/2
  Product/1 -> Add/5
  Product2/1 -> Add/6
  Bus Selector/7 -> [Rudder]  "<Rudder>"
  Bus Selector/3 -> [P]  "<P>"
  Bus Selector/5 -> [HorizontalTail]  "<Horizontal Tail>"
  States/1 -> Bus Selector/1
  Bus Selector/2 -> [Beta]  "<Beta>"
  Bus Selector/10 -> [Velocity]  "<Velocity>"
  Bus Selector/1 -> [Alpha]  "<Alpha>"
  Bus Selector/6 -> [Aileron]  "<Aileron>"
  Bus Selector/8 -> [LeadingEdgeFlap]  "<LEF>"
  Bus Selector/4 -> [R]  "<R>"
  Bus Selector/9 -> Terminator/1  "<Speed Brake>"
  Wing Span1/1 -> Sum8/1
  Sum8/1 -> [LeadingEdgeFlapDeflectionDelta]

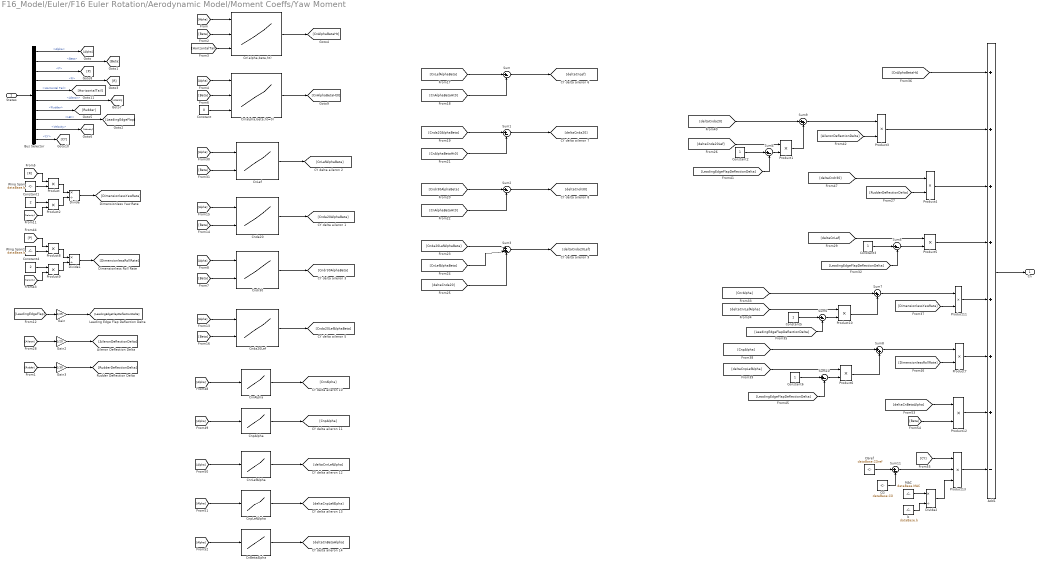
== system F16_Model/Euler/F16 Euler Rotation/Aerodynamic Model/Moment Coeffs/Yaw Moment ==
  States : Inport
  Add1 : Sum  Inputs=+++++++-
  Bus Selector : BusSelector  OutputSignals=Alpha,Beta,P,R,Horizontal Tail,Aileron,Rudder,LEF,Velocity,CY
  CG : Constant  Value=dataBase.CG
  CGref : Constant  Value=dataBase.CGref
  Cn(alpha,beta,ht) : Lookup_n-D  NumberOfTableDimensions=3  BreakpointsForDimension1=dataBase.f16_AerodynamicData.BP.Cn.Cn.alpha  BreakpointsForDimension2=dataBase.f16_AerodynamicData.BP.Cn.Cn.beta  BreakpointsForDimension3=dataBase.f16_AerodynamicData.BP.Cn.Cn.dHT  Table=dataBase.f16_AerodynamicData.data.Cn.Cn  ExtrapMethod=Clip  InternalRulePriority=Speed  RndMeth=Simplest
      settings: InputPortMap=u0,u1,u2
  Cn(alpha,beta,ht=0) : Lookup_n-D  NumberOfTableDimensions=3  BreakpointsForDimension1=dataBase.f16_AerodynamicData.BP.Cn.Cn.alpha  BreakpointsForDimension2=dataBase.f16_AerodynamicData.BP.Cn.Cn.beta  BreakpointsForDimension3=dataBase.f16_AerodynamicData.BP.Cn.Cn.dHT  Table=dataBase.f16_AerodynamicData.data.Cn.Cn  ExtrapMethod=Clip  InternalRulePriority=Speed  RndMeth=Simplest
      settings: InputPortMap=u0,u1,u2
  CnBetaAlpha : Lookup_n-D  NumberOfTableDimensions=1  BreakpointsForDimension1=dataBase.f16_AerodynamicData.BP.Cn.deltaCnBeta.alpha  Table=dataBase.f16_AerodynamicData.data.Cn.deltaCnBeta  ExtrapMethod=Clip  InternalRulePriority=Speed  RndMeth=Simplest
  CnLef : Lookup_n-D  BreakpointsForDimension1=dataBase.f16_AerodynamicData.BP.Cn.Cnlef.alpha  BreakpointsForDimension2=dataBase.f16_AerodynamicData.BP.Cn.Cnlef.beta  Table=dataBase.f16_AerodynamicData.data.Cn.Cnlef  ExtrapMethod=Clip  InternalRulePriority=Speed  RndMeth=Simplest
      settings: InputPortMap=u0,u1
  Cnda20 : Lookup_n-D  BreakpointsForDimension1=dataBase.f16_AerodynamicData.BP.Cn.Cnda20.alpha  BreakpointsForDimension2=dataBase.f16_AerodynamicData.BP.Cn.Cnda20.beta  Table=dataBase.f16_AerodynamicData.data.Cn.Cnda20  ExtrapMethod=Clip  InternalRulePriority=Speed  RndMeth=Simplest
      settings: InputPortMap=u0,u1
  Cnda20Lef : Lookup_n-D  BreakpointsForDimension1=dataBase.f16_AerodynamicData.BP.Cn.Cnda20lef.alpha  BreakpointsForDimension2=dataBase.f16_AerodynamicData.BP.Cn.Cnda20lef.beta  Table=dataBase.f16_AerodynamicData.data.Cn.Cnda20lef  ExtrapMethod=Clip  InternalRulePriority=Speed  RndMeth=Simplest
      settings: InputPortMap=u0,u1
  Cndr30 : Lookup_n-D  BreakpointsForDimension1=dataBase.f16_AerodynamicData.BP.Cn.Cndr30.alpha  BreakpointsForDimension2=dataBase.f16_AerodynamicData.BP.Cn.Cndr30.beta  Table=dataBase.f16_AerodynamicData.data.Cn.Cndr30  ExtrapMethod=Clip  InternalRulePriority=Speed  RndMeth=Simplest
      settings: InputPortMap=u0,u1
  CnpAlpha : Lookup_n-D  NumberOfTableDimensions=1  BreakpointsForDimension1=dataBase.f16_AerodynamicData.BP.Cn.Cnp.alpha  Table=dataBase.f16_AerodynamicData.data.Cn.Cnp  ExtrapMethod=Clip  InternalRulePriority=Speed  RndMeth=Simplest
  CnpLefAlpha : Lookup_n-D  NumberOfTableDimensions=1  BreakpointsForDimension1=dataBase.f16_AerodynamicData.BP.Cn.deltaCnplef.alpha  Table=dataBase.f16_AerodynamicData.data.Cn.deltaCnplef  ExtrapMethod=Clip  InternalRulePriority=Speed  RndMeth=Simplest
  CnrAlpha : Lookup_n-D  NumberOfTableDimensions=1  BreakpointsForDimension1=dataBase.f16_AerodynamicData.BP.Cn.Cnr.alpha  Table=dataBase.f16_AerodynamicData.data.Cn.Cnr  ExtrapMethod=Clip  InternalRulePriority=Speed  RndMeth=Simplest
  CnrLefAlpha : Lookup_n-D  NumberOfTableDimensions=1  BreakpointsForDimension1=dataBase.f16_AerodynamicData.BP.Cn.deltaCnrlef.alpha  Table=dataBase.f16_AerodynamicData.data.Cn.deltaCnrlef  ExtrapMethod=Clip  InternalRulePriority=Speed  RndMeth=Simplest
  Constant : Constant  Value=0
  Constant1 : Constant  Value=2
  Constant{2..3,5..6} (4 alike) : Constant
  Constant4 : Constant  Value=2
  Divide : Product  Inputs=*/
  Divide1 : Product  Inputs=*/
  Divide2 : Product  Inputs=*/
  Gain : Gain  Gain=1/25
  Gain2 : Gain  Gain=1/20
  Gain3 : Gain  Gain=1/30
  MAC : Constant  Value=dataBase.MAC
  Product{,1..12} (13 alike) : Product
  Product13 : Product  Inputs=3
  Sum{,1..2,4..6,10..11} (8 alike) : Sum  Inputs=|+-
  Sum3 : Sum  Inputs=|+--
  Sum7 : Sum  Inputs=|++
  Sum8 : Sum  Inputs=|++
  Sum9 : Sum  Inputs=|++
  Wing Span : Constant  Value=dataBase.b
  Wing Span1 : Constant  Value=dataBase.b
  b : Constant  Value=dataBase.b
  Cn : Outport
  wires:
  States/1 -> Bus Selector/1
  [Velocity] -> Product2/2
  Product2/1 -> Divide/2
  [R] -> Product/1
  Constant1/1 -> Product2/1
  Wing Span/1 -> Product/2
  Wing Span1/1 -> Product8/2
  [P] -> Product8/1
  Constant4/1 -> Product9/1
  Product8/1 -> Divide1/1
  Divide1/1 -> [DimensionlessRollRate]
  Product9/1 -> Divide1/2
  Divide/1 -> [DimensionlessYawRate]
  Product/1 -> Divide/1
  [Velocity] -> Product9/2
  [LeadingEdgeFlap] -> Gain/1
  Gain2/1 -> [AileronDeflectionDelta]
  [Aileron] -> Gain2/1
  [Rudder] -> Gain3/1
  Gain3/1 -> [RudderDeflectionDelta]
  Gain/1 -> [LeadingEdgeFlapDeflectionDelta]
  [HorizontalTail] -> Cn(alpha,beta,ht)/3
  [Alpha] -> Cn(alpha,beta,ht)/1
  [Beta] -> Cn(alpha,beta,ht)/2
  Cn(alpha,beta,ht)/1 -> [CnAlphaBetaHt]
  Cn(alpha,beta,ht=0)/1 -> [CnAlphaBetaHt0]
  [Beta] -> Cn(alpha,beta,ht=0)/2
  [Alpha] -> Cn(alpha,beta,ht=0)/1
  Constant/1 -> Cn(alpha,beta,ht=0)/3
  [Beta] -> CnLef/2
  CnLef/1 -> [CnLefAlphaBeta]
  [Alpha] -> CnLef/1
  [Alpha] -> Cnda20/1
  [Beta] -> Cnda20/2
  Cnda20/1 -> [Cnda20AlphaBeta]
  Cndr30/1 -> [Cndr30AlphaBeta]
  [Beta] -> Cndr30/2
  [Alpha] -> Cndr30/1
  Cnda20Lef/1 -> [Cnda20LefAlphaBeta]
  [Beta] -> Cnda20Lef/2
  [Alpha] -> Cnda20Lef/1
  [CnLefAlphaBeta] -> Sum/1
  [CnAlphaBetaHt0] -> Sum/2
  Sum/1 -> [deltaCnLef]
  Sum1/1 -> [deltaCnda20]
  [CnAlphaBetaHt0] -> Sum1/2
  [Cnda20AlphaBeta] -> Sum1/1
  [Cndr30AlphaBeta] -> Sum2/1
  [CnAlphaBetaHt0] -> Sum2/2
  Sum2/1 -> [deltaCndr30]
  [Cnda20LefAlphaBeta] -> Sum3/1
  [CnLefAlphaBeta] -> Sum3/2
  [deltaCnda20] -> Sum3/3
  Sum3/1 -> [deltaCnda20Lef]
  Product5/1 -> Add1/4
  Add1/1 -> Cn/1
  [LeadingEdgeFlapDeflectionDelta] -> Sum10/2
  [LeadingEdgeFlapDeflectionDelta] -> Sum5/2
  Sum10/1 -> Product6/2
  [deltaCnLef] -> Product5/1
  [LeadingEdgeFlapDeflectionDelta] -> Sum6/2
  Constant6/1 -> Sum10/1
  Constant5/1 -> Sum6/1
  Product1/1 -> Sum9/2
  [CnpAlpha] -> Sum8/1
  Product6/1 -> Sum8/2
  Sum5/1 -> Product5/2
  [deltaCnrLefAlpha] -> Product10/1
  Product4/1 -> Add1/3
  Constant2/1 -> Sum4/1
  [deltaCnpLefAlpha] -> Product6/1
  Sum4/1 -> Product1/2
  [LeadingEdgeFlapDeflectionDelta] -> Sum4/2
  Product7/1 -> Add1/6
  [DimensionlessYawRate] -> Product11/2
  Constant3/1 -> Sum5/1
  [DimensionlessRollRate] -> Product7/2
  Sum7/1 -> Product11/1
  Sum8/1 -> Product7/1
  Product11/1 -> Add1/5
  [CnrAlpha] -> Sum7/1
  [deltaCndr30] -> Product4/1
  Product10/1 -> Sum7/2
  Sum9/1 -> Product3/1
  Product3/1 -> Add1/2
  [deltaCnda20] -> Sum9/1
  Sum6/1 -> Product10/2
  [RudderDeflectionDelta] -> Product4/2
  [deltaCnda20Lef] -> Product1/1
  [CnAlphaBetaHt] -> Add1/1
  [AileronDeflectionDelta] -> Product3/2
  CnrAlpha/1 -> [CnrAlpha]
  [Alpha] -> CnrAlpha/1
  [Alpha] -> CnpAlpha/1
  CnpAlpha/1 -> [CnpAlpha]
  CnpLefAlpha/1 -> [deltaCnpLefAlpha]
  [Alpha] -> CnpLefAlpha/1
  [Alpha] -> CnrLefAlpha/1
  CnrLefAlpha/1 -> [deltaCnrLefAlpha]
  [Alpha] -> CnBetaAlpha/1
  CnBetaAlpha/1 -> [deltaCnBetaAlpha]
  [deltaCnBetaAlpha] -> Product12/1
  [Beta] -> Product12/2
  Product12/1 -> Add1/7
  CGref/1 -> Sum11/1
  Sum11/1 -> Product13/2
  CG/1 -> Sum11/2
  b/1 -> Divide2/2
  MAC/1 -> Divide2/1
  Divide2/1 -> Product13/3
  [CY] -> Product13/1
  Product13/1 -> Add1/8
  Bus Selector/1 -> [Alpha]  "<Alpha>"
  Bus Selector/2 -> [Beta]  "<Beta>"
  Bus Selector/4 -> [R]  "<R>"
  Bus Selector/3 -> [P]  "<P>"
  Bus Selector/5 -> [HorizontalTail]  "<Horizontal Tail>"
  Bus Selector/6 -> [Aileron]  "<Aileron>"
  Bus Selector/7 -> [Rudder]  "<Rudder>"
  Bus Selector/8 -> [LeadingEdgeFlap]  "<LEF>"
  Bus Selector/9 -> [Velocity]  "<Velocity>"
  Bus Selector/10 -> [CY]  "<CY>"

== matlab function F16_Model/Euler/F16 Euler Rotation/Atmosphere Model/MATLAB Function ==
  data: h input; g output; V input; T output; P output; rho output; Qdyn output; M output
%% Atmospheric Model

function [g,T,P,rho,Qdyn,M] = fcn(h,V)

g = 9.80665*(6371020/(6371020+h))^2;
T = 288.15 - 6.5*h/1000;
P = 101325*(T/288.15)^(g/1.86584);
rho = P/(287.053*T);
k = 1.4;
R_c = 287.06;
M = V/sqrt(k*R_c*T);
Qdyn = 0.5*rho*V^2;

== matlab function F16_Model/Euler/F16 Euler Rotation/Equations of Motion Block/F16 EoM ==
  data: Forces input size=3; Moments input size=3; Thrust input size=4; Mass_Inertia input; Gravity input; xDot output size=12; states input size=12; loadsBody output size=3
function [xDot, loadsBody]  = fcn(Forces, Moments, Thrust, Mass_Inertia, Gravity, states)

Alpha = states(1);
Beta = states(2);
Theta = states(3);
Phi = states(4);
Psi = states(5);
P = states(6);
Q = states(7);
R = states(8);
Velocity = states(9);
North = states(10);
East = states(11);
Altitude = states(12);

g = Gravity;

%% --------------- Forces on the Body of the Aircraft -------- %%

% Aerodynamic Forces and Moments
Fx = Forces(1);
Fy = Forces(2);
Fz = Forces(3);

Gyro_moment = [Thrust(2); Thrust(3); Thrust(4)];

pitchingMoment = Moments(1) + Gyro_moment(2); % M
rollingMoment = Moments(2) + Gyro_moment(1); % L
yawingMoment = Moments(3) + Gyro_moment(3); % N

% Thrust Forces
Thrust_x = Thrust(1);
Thrust_y = 0;
Thrust_z = 0;

% Gravitational Forces
Fg_body = Mass_Inertia(6);

% Total Forces
Fx_total = Fx + Thrust_x;
Fy_total = Fy + Thrust_y;
Fz_total = Fz + Thrust_z;

Nx = Fx_total/(Mass_Inertia(1)*g);
Ny = Fy_total/(Mass_Inertia(1)*g);
Nz = -Fz_total/(Mass_Inertia(1)*g);

loadsBody = [Nx; Ny; Nz];

F_total = [Fx_total; Fy_total; Fz_total] + Fg_body;

%% Forces in Wind Frame

transFromBtoW = [cos(Beta)*cos(Alpha) sin(Beta) cos(Beta)*sin(Alpha);...
                 -sin(Beta)*cos(Alpha) cos(Beta) -sin(Beta)*sin(Alpha);...
                 -sin(Alpha) 0 cos(Alpha)];
        
forceCoeffsBody = [Fx; Fy; Fz];
forceCoeffsWind = transFromBtoW*forceCoeffsBody;

D = -forceCoeffsWind(1);
Y = forceCoeffsWind(2);
L = -forceCoeffsWind(3);

%% ---------------- Mass and Inertia Properties ------------------ %%

Mass = Mass_Inertia(1); % kg
Ixx = Mass_Inertia(2); % kgm^2
Iyy = Mass_Inertia(3); % kgm^2
Izz = Mass_Inertia(4); % kgm^2
Ixz = Mass_Inertia(5); % kgm^2

%% ---------------- Propagation of States ------------------------- %%

%% Equations of Motion

% Translational Eq.s of Motion
U = Velocity*cos(Alpha)*cos(Beta);
V = Velocity*sin(Beta);
W = Velocity*sin(Alpha)*cos(Beta);
% 
% UDot = R*V - Q*W + Fg_body(1) + Fx_total/Mass;
% VDot = P*W - R*U + Fg_body(2) + Fy_total/Mass;
% WDot = Q*U - P*V + Fg_body(3) + Fz_total/Mass;

% Rotational Eq.s of Motion
F = Ixx*Izz - Ixz^2;
PDot = (Ixz*(Ixx-Iyy+Izz)*P*Q - (Izz*(Izz-Iyy)+Ixz^2)*Q*R + Izz*rollingMoment + Ixz*yawingMoment)/F;
QDot = ((Izz-Ixx)*P*R - Ixz*(R^2 - P^2) + pitchingMoment)/Iyy;
RDot = ((Ixx*(Ixx-Iyy)+Ixz^2)*P*Q - Ixz*(Ixx-Iyy+Izz)*Q*R + Ixz*rollingMoment + Ixx*yawingMoment)/F;

% Kinematic Eq.s
ThetaDot = Q*cos(Phi) - R*sin(Phi);
PhiDot = P + tan(Theta)*(Q*sin(Phi) + R*cos(Phi));
PsiDot = (Q*sin(Phi) + R*cos(Phi))/cos(Theta);

% Navigational Eq.s 
NorthDot = U*cos(Theta)*cos(Psi) + V*(-cos(Phi)*sin(Psi) + sin(Phi)*sin(Theta)*cos(Psi)) ...
                                        + W*(sin(Phi)*sin(Psi)+cos(Phi)*sin(Theta)*cos(Psi));
EastDot = U*cos(Theta)*sin(Psi) +  V*(cos(Phi)*cos(Psi) + sin(Phi)*sin(Theta)*sin(Psi)) ...
                                     + W*(-sin(Phi)*cos(Psi) + cos(Phi)*sin(Theta)*sin(Psi));
AltitudeDot = Velocity*(cos(Alpha)*cos(Beta)*sin(Theta) - sin(Beta)*sin(Phi)*cos(Theta)...
                                            - sin(Alpha)*cos(Beta)*cos(Phi)*cos(Theta));

% Auxiliary
AlphaDot = (-L - Thrust_x*sin(Alpha))/(Mass*Velocity*cos(Beta)) + g*(cos(Theta)*cos(Phi)*cos(Alpha)...
    + sin(Theta)*sin(Alpha))/(Velocity*cos(Beta)) + Q - tan(Beta)*(P*cos(Alpha) + R*sin(Alpha));

BetaDot = (D*sin(Beta)+Y*cos(Beta) - Thrust_x*cos(Alpha)*sin(Beta))/(Mass*Velocity)...
    + g*(sin(Theta)*cos(Alpha)*sin(Beta) + cos(Theta)*sin(Phi)*cos(Beta)...
    - cos(Theta)*cos(Phi)*sin(Alpha)*sin(Beta))/Velocity + P*sin(Alpha) - R*cos(Alpha);

VelocityDot = (-D*cos(Beta) + Y*sin(Beta) + Thrust_x*cos(Alpha)*cos(Beta))/Mass + ...
                g*(-sin(Theta)*cos(Alpha)*cos(Beta) +...
                cos(Theta)*sin(Phi)*sin(Beta) + cos(Theta)*cos(Phi)*sin(Alpha)*cos(Beta));
            
           
xDot = [AlphaDot, BetaDot, ThetaDot, PhiDot, PsiDot, PDot, QDot, RDot, ...
                                    VelocityDot, NorthDot, EastDot, AltitudeDot]';

== matlab function F16_Model/Euler/F16 Euler Rotation/Mass & Inertia/MATLAB Function ==
  data: g input; Mass output; theta input; Ixx output; Iyy output; Izz output; Ixz output; phi input; Fg_body output
function [Mass,Ixx,Iyy ,Izz,Ixz,Fg_body] = fcn(g,theta,phi)

%% Mass
Mass = 91188/9.8065; % kg

%% Moments of Inertia
Ixx = 12875; % kgm^2
Iyy = 75674; % kgm^2
Izz = 85552; % kgm^2
Ixz = 1331; % kgm^2

%% Gravitational Forces in Body Frame

Fg_body = [ -Mass*g*sin(theta); 
             Mass*g*cos(theta)*sin(phi);
             Mass*g*cos(theta)*cos(phi)];

== matlab function F16_Model/Euler/F16 Euler Rotation/Propulsion Model/MATLAB Function1 ==
  data: Tidle input size=1; Thrust output size=1; Tmil input size=1; Tmax input size=1; Throttle input size=1
function Thrust = fcn(Tidle, Tmil, Tmax, Throttle)

if Throttle <= 77
    Pc = 64.94*Throttle/100;
elseif Throttle > 77
    Pc = 217.38*Throttle/100 - 117.38;
else
    Pc = 0;
end

if Pc < 50
    Thrust = Tidle + (Tmil - Tidle)*Pc/50;
elseif 50 <= Pc
    Thrust = Tmil + (Tmax - Tmil)*(Pc-50)/50;
else
    Thrust = 0;
end

== matlab function F16_Model/Euler/F16 Euler Rotation/Propulsion Model/MATLAB Function ==
  data: Q input; T_moment output; R input




function T_moment = fcn(Q,R)

He = 216.9;

T_moment = [0 ; -He*R; He*Q];
